simulink model "lab6fsf_nonlinear"  (R2024a)
settings: Solver=ode45  StartTime=0.0  StopTime=20.0  RelTol=1e-3
values from neighbouring files (symbols this model uses):
  k1 = lqr(A,B,Q,R)    [ica19_runscript.m]
  x0 = [0;0;5/180*pi;0]    [ica19_runscript.m]
  xs = [0;0;0;0]    [ica19_runscript.m]
settings Model: Creator=Lauren  LastModifiedBy=Lauren
settings DataIOCC: SaveOutput=off  SignalLogging=off  DSMLogging=off  SaveTime=off  ReturnWorkspaceOutputs=off

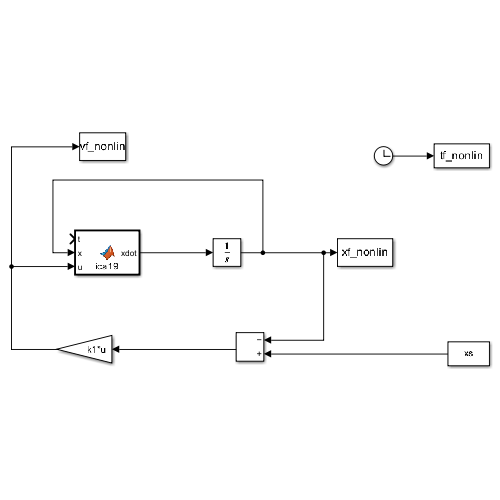
[thumbnail: Simulink's stored preview of the top-level diagram]
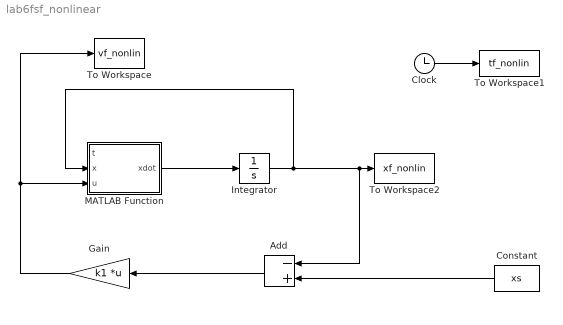
== system lab6fsf_nonlinear ==
  Add : Sum  Inputs=-+
  Clock : Clock
  Constant : Constant  Value=xs
  Gain : Gain  Gain=k1  Multiplication=Matrix(K*u)
  Integrator : Integrator  InitialCondition=x0
  MATLAB Function : MATLAB Function  TreatAsAtomicUnit=on
  To Workspace : ToWorkspace  VariableName=vf_nonlin  SampleTime=-1
      settings: Save2DSignal=2-D array (concatenate along first dimension)
  To Workspace1 : ToWorkspace  VariableName=tf_nonlin  SampleTime=-1
      settings: Save2DSignal=2-D array (concatenate along first dimension)
  To Workspace2 : ToWorkspace  VariableName=xf_nonlin  SampleTime=-1
      settings: Save2DSignal=2-D array (concatenate along first dimension)
  wires:
  Clock/1 -> To Workspace1/1
  Integrator/1 -> Add/1, To Workspace2/1, MATLAB Function/2(x)
  Add/1 -> Gain/1
  Constant/1 -> Add/2
  Gain/1 -> MATLAB Function/3(u), To Workspace/1
  MATLAB Function/1(xdot) -> Integrator/1

== matlab function lab6fsf_nonlinear/MATLAB Function ==
  data: t input; x input; u input; xdot output
function xdot  = ica19(t,x,u)

xdot = ica19(t,x,u);
